simulink model "Inverter1"  (Simulink 10.0)
settings: Solver=ode23tb  StartTime=0.0  StopTime=5  RelTol=1e-3  EnableMultiTasking=on
libraries: powerlib x12
Description:
  | Single Phase Full Bridge Inverter
  | Input is through Dc voltage source.
  | Output can be seen at the load.
  | When Gto1 & Gto3 conducts load voltage is equal to dc voltage source.
  | When Gto2 & Gto4 conducts load voltage is equal to negarive of dc voltage source.
settings Model: Creator=Shailesh  LastModifiedBy=bhisma
settings DataIOCC: LimitDataPoints=on  SignalLoggingSaveFormat=ModelDataLogs
settings OptimizationCC: ExpressionDepthLimit=2147483647  InitFltsAndDblsToZero=on
settings DebuggingCC: SaveWithParameterizedLinksMsg=none  SignalResolutionControl=TryResolveAllWithWarning  SolverPrmCheckMsg=warning  MultiTaskDSMMsg=warning  MultiTaskCondExecSysMsg=none  FcnCallInpInsideContextMsg=warning  StateNameClashWarn=warning
settings GRTTargetCC: TargetFcnLib=ansi_tfl_tmw.mat  GeneratePreprocessorConditionals=Disable all
settings ConfigComp: CovExternalEMLEnable=off

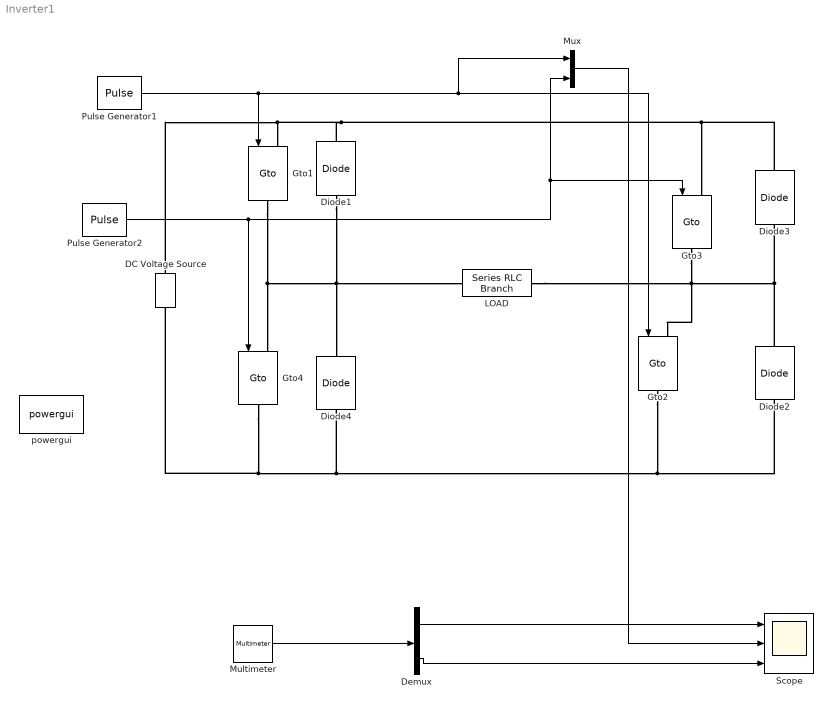
== system Inverter1 ==
  DC Voltage Source : powerlib/Electrical Sources/DC Voltage Source  SystemSampleTime=-1  Amplitude=5  Measurements=Voltage
      settings: SourceProductName=Simscape Electrical
  Demux : Demux  Outputs=2
  Diode{1..4} (4 alike) : powerlib/Power Electronics/Diode  SystemSampleTime=-1  Ron=0.001  Lon=0  Vf=0  IC=0  UseSnubber=off  Rs=500  Cs=250e-9  Measurements=off
      settings: SourceProductName=Simscape Electrical
  Gto{1..4} (4 alike) : powerlib/Power Electronics/Gto  SystemSampleTime=-1  Ron=0.001  Lon=1e-6  Vf=0  Tf=10e-6  Tt=20e-6  IC=0  Rs=1e5  Cs=inf  Measurements=off
      settings: SourceProductName=Simscape Electrical  SourceProductBaseCode=PS
  LOAD : powerlib/Elements/Series RLC Branch  PhysicalDomain=powersysdomain  SubClassName=unknown  LeftPortType=p1  RightPortType=p1  LConnTagsString=__new0  RConnTagsString=__new0  BranchType=RLC  Resistance=1  Inductance=0  SetiL0=off  InitialCurrent=0  Capacitance=inf  Setx0=off  InitialVoltage=0  Measurements=Branch voltage
      settings: SourceProductName=Simscape Electrical
  Multimeter : powerlib/Measurements/Multimeter  SystemSampleTime=-1  PhasorSimulation=off  OutputType=Complex  sel=[2 1]  L=2  Gain=[1 1]  yselected={'Usrc: DC Voltage Source','Ub: LOAD'};  PSBOutputType=1  PSBequivalent=0  AxesSetting=[0,0.1,-100,100]  Display=0  SavedBlockNames=-11
      settings: SourceProductName=Simscape Electrical
  Mux : Mux  Inputs=2
  Pulse Generator1 : DiscretePulseGenerator  PulseType=Time based  Period=1  PulseWidth=50
  Pulse Generator2 : DiscretePulseGenerator  PulseType=Time based  Period=1  PulseWidth=50  PhaseDelay=0.5
  Scope : Scope  NumInputPorts=3
  powergui : powerlib/powergui  Priority=1  SystemSampleTime=-1  SimulationMode=Continuous  SampleTime=50e-6  frequency=60  SPID=off  DisableSnubberDevices=off  DisableRonSwitches=off  DisableVfSwitches=off  SwTol=0  Interpol=off  DisplayEquations=off  FunctionMessages=off  frequencyindice=0  Pbase=100e6  ErrMax=1e-4  Iterations=50  UnitsV=kV  UnitsW=MW  echomessages=off  HookPort=off  EnableUseOfTLC=off  x0status=blocks  RestoreLinks=warning  ResistiveCurrentMeasurement=off  Frange=[0:2:500]  Ylog=off  Xlog=on  ShowGrid=off  save=off  variable=ZData  ZoomFFT=off  StartTime=0.0  cycles=1  DisplayStyle=1  FreqAxis=off  MaxFrequency=1000  frequencyindicesteady=1  display=off  methode=off
      settings: SourceProductName=Simscape Electrical
  wires:
  Multimeter/1 -> Demux/1
  Pulse Generator1/1 -> Gto1/1, Gto2/1, Mux/1
  Pulse Generator2/1 -> Gto4/1, Gto3/1, Mux/2
  Demux/1 -> Scope/1
  Mux/1 -> Scope/2
  Demux/2 -> Scope/3
  connections:
  Gto1/RConn1 -- Diode1/LConn1 -- Diode4/RConn1 -- LOAD/LConn1 -- Gto4/LConn1
  Gto4/RConn1 -- Diode4/LConn1 -- Diode2/LConn1 -- Gto2/RConn1 -- DC Voltage Source/LConn1
  Diode1/RConn1 -- Diode3/RConn1 -- Gto3/LConn1 -- Gto1/LConn1 -- DC Voltage Source/RConn1
  LOAD/RConn1 -- Gto3/RConn1 -- Gto2/LConn1 -- Diode3/LConn1 -- Diode2/RConn1
